simulink model "Drone2_simulink_old"  (R2024b)
settings: Solver=ode1be  StartTime=0.0  StopTime=1200  FixedStep=0.001  MaxStep=0.001  MinStep=0.00095  RelTol=1e-3
undefined symbols (not defined in the file): DiscIntNeverNeededParam, Environment, Newton, Raphson, Sim3dSensor, Vehicle, X, Y, Z
libraries: sm_lib x2953, nesl_utility x76, slpidlib x25, simulink x4, eeGeneralControl x4, matrix_library x3, rllib x2, sim3dlib x2, uavsim3dlib x2, dspstat3 x1, SignalEditorBlockLib x1, sharedutil x1
(part 6 of 21)

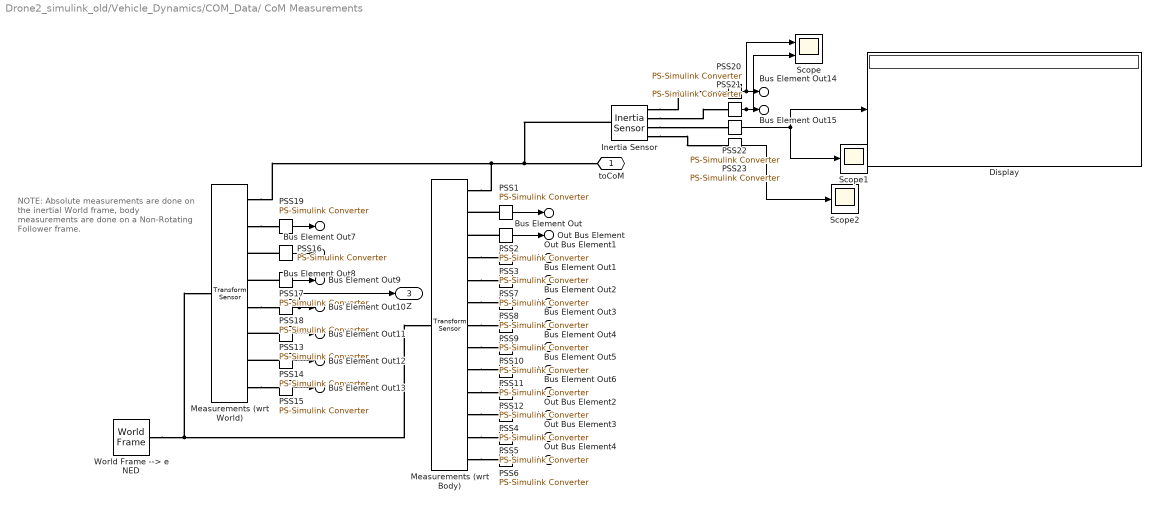
== system Drone2_simulink_old/Vehicle_Dynamics/COM_Data/ CoM Measurements ==
  note: NOTE:
      | Absolute measurements are done on the inertial World frame, body measurements are done on a Non-Rotating Follower frame.
  Display : Display
  Inertia Sensor : sm_lib/Body Elements/Inertia Sensor  SensorExtent=BodyGroup  SpanWeldJoints=off  ExcludeGroundedBodies=off  MeasurementFrame=Attached  SenseMass=on  SenseCenterOfMass=on  SenseInertiaMatrix=on  SenseCenteredInertiaMatrix=off  SensePrincipalInertiaMatrix=on  SenseRotationMatrix=off  GraphicType=PrincipalInertiaFrame  PrincipalInertiaFrameSize=20  GraphicVisPropType=SimpleVisualProperties  GraphicDiffuseColor=[1 0 1]  GraphicOpacity=1  GraphicSpecularColor=[0.5 0.5 0.5 1.0]  GraphicAmbientColor=[0.15 0.15 0.15 1.0]  GraphicEmissiveColor=[0.0 0.0 0.0 1.0]  GraphicShininess=75
  Measurements (wrt Body) : sm_lib/Frames and Transforms/Transform Sensor  MeasurementFrame=NonRotatingFollower  RotationSequence=ZYX  SenseAngle=off  SenseAxis=off  SenseQ=off  SenseR=off  SenseRotationSequence=off  SenseOmegaX=on  SenseOmegaY=on  SenseOmegaZ=on  SenseOmega=off  SenseQDot=off  SenseRDot=off  SenseRotationSequenceDot=off  SenseAlphaX=on  SenseAlphaY=on  SenseAlphaZ=on  SenseAlpha=off  SenseQDDot=off  SenseRDDot=off  SenseX=off  SenseY=off  SenseZ=off  SenseXYZ=off  SenseRad=off  SenseAzim=off  SenseDist=off  SenseInc=off  SenseXDot=on  SenseYDot=on  SenseZDot=on  SenseXYZDot=off  SenseRadDot=off  SenseAzimDot=off  SenseDistDot=off  SenseIncDot=off  SenseXDDot=on  SenseYDDot=on  SenseZDDot=on  SenseXYZDDot=off  SenseRadDDot=off  SenseAzimDDot=off  SenseDistDDot=off  SenseIncDDot=off
  Measurements (wrt World) : sm_lib/Frames and Transforms/Transform Sensor  MeasurementFrame=World  RotationSequence=ZYX  SenseAngle=off  SenseAxis=off  SenseQ=off  SenseR=on  SenseRotationSequence=off  SenseOmegaX=off  SenseOmegaY=off  SenseOmegaZ=off  SenseOmega=off  SenseQDot=off  SenseRDot=off  SenseRotationSequenceDot=off  SenseAlphaX=off  SenseAlphaY=off  SenseAlphaZ=off  SenseAlpha=off  SenseQDDot=off  SenseRDDot=off  SenseX=on  SenseY=on  SenseZ=on  SenseXYZ=off  SenseRad=off  SenseAzim=off  SenseDist=off  SenseInc=off  SenseXDot=on  SenseYDot=on  SenseZDot=on  SenseXYZDot=off  SenseRadDot=off  SenseAzimDot=off  SenseDistDot=off  SenseIncDot=off  SenseXDDot=off  SenseYDDot=off  SenseZDDot=off  SenseXYZDDot=off  SenseRadDDot=off  SenseAzimDDot=off  SenseDistDDot=off  SenseIncDDot=off
  PSS1 : nesl_utility/PS-Simulink Converter  PhysicalDomain=network_engine_domain  SubClassName=ps_output  LeftPortType=input  RightPortType=output  PseudoPeriodic=off  Frequencies=[]  VectorFormat=1-D array  Unit=rad/s  AffineConversion=off
  PSS{10..15} (6 alike) : nesl_utility/PS-Simulink Converter  PhysicalDomain=network_engine_domain  SubClassName=ps_output  LeftPortType=input  RightPortType=output  PseudoPeriodic=off  Frequencies=[]  VectorFormat=1-D array  Unit=m/s  AffineConversion=off
  PSS{16..18,21} (4 alike) : nesl_utility/PS-Simulink Converter  PhysicalDomain=network_engine_domain  SubClassName=ps_output  LeftPortType=input  RightPortType=output  PseudoPeriodic=off  Frequencies=[]  VectorFormat=1-D array  Unit=m  AffineConversion=off
  PSS19 : nesl_utility/PS-Simulink Converter  PhysicalDomain=network_engine_domain  SubClassName=ps_output  LeftPortType=input  RightPortType=output  PseudoPeriodic=off  Frequencies=[]  VectorFormat=1-D array  Unit=1  AffineConversion=off
  PSS2 : nesl_utility/PS-Simulink Converter  PhysicalDomain=network_engine_domain  SubClassName=ps_output  LeftPortType=input  RightPortType=output  PseudoPeriodic=off  Frequencies=[]  VectorFormat=1-D array  Unit=rad/s  AffineConversion=off
  PSS20 : nesl_utility/PS-Simulink Converter  PhysicalDomain=network_engine_domain  SubClassName=ps_output  LeftPortType=input  RightPortType=output  PseudoPeriodic=off  Frequencies=[]  VectorFormat=1-D array  Unit=kg  AffineConversion=off
  PSS22 : nesl_utility/PS-Simulink Converter  PhysicalDomain=network_engine_domain  SubClassName=ps_output  LeftPortType=input  RightPortType=output  PseudoPeriodic=off  Frequencies=[]  VectorFormat=1-D array  Unit=1  AffineConversion=on
  PSS23 : nesl_utility/PS-Simulink Converter  PhysicalDomain=network_engine_domain  SubClassName=ps_output  LeftPortType=input  RightPortType=output  PseudoPeriodic=off  Frequencies=[]  VectorFormat=1-D array  Unit=1  AffineConversion=on
  PSS3 : nesl_utility/PS-Simulink Converter  PhysicalDomain=network_engine_domain  SubClassName=ps_output  LeftPortType=input  RightPortType=output  PseudoPeriodic=off  Frequencies=[]  VectorFormat=1-D array  Unit=rad/s  AffineConversion=off
  PSS4 : nesl_utility/PS-Simulink Converter  PhysicalDomain=network_engine_domain  SubClassName=ps_output  LeftPortType=input  RightPortType=output  PseudoPeriodic=off  Frequencies=[]  VectorFormat=1-D array  Unit=m/s^2  AffineConversion=off
  PSS5 : nesl_utility/PS-Simulink Converter  PhysicalDomain=network_engine_domain  SubClassName=ps_output  LeftPortType=input  RightPortType=output  PseudoPeriodic=off  Frequencies=[]  VectorFormat=1-D array  Unit=m/s^2  AffineConversion=off
  PSS6 : nesl_utility/PS-Simulink Converter  PhysicalDomain=network_engine_domain  SubClassName=ps_output  LeftPortType=input  RightPortType=output  PseudoPeriodic=off  Frequencies=[]  VectorFormat=1-D array  Unit=m/s^2  AffineConversion=off
  PSS7 : nesl_utility/PS-Simulink Converter  PhysicalDomain=network_engine_domain  SubClassName=ps_output  LeftPortType=input  RightPortType=output  PseudoPeriodic=off  Frequencies=[]  VectorFormat=1-D array  Unit=rad/s^2  AffineConversion=off
  PSS8 : nesl_utility/PS-Simulink Converter  PhysicalDomain=network_engine_domain  SubClassName=ps_output  LeftPortType=input  RightPortType=output  PseudoPeriodic=off  Frequencies=[]  VectorFormat=1-D array  Unit=rad/s^2  AffineConversion=off
  PSS9 : nesl_utility/PS-Simulink Converter  PhysicalDomain=network_engine_domain  SubClassName=ps_output  LeftPortType=input  RightPortType=output  PseudoPeriodic=off  Frequencies=[]  VectorFormat=1-D array  Unit=rad/s^2  AffineConversion=off
  Scope : Scope  NumInputPorts=2
  Scope1 : Scope
  Scope2 : Scope
  World Frame --> e NED : sm_lib/Frames and Transforms/World Frame
  toCoM : PMIOPort  Side=Left
  Bus Element Out : Outport  PortName=Body  Element=wb.p
  Out Bus Element : Outport  PortName=Body  Element=wb.q
  Out Bus Element1 : Outport  PortName=Body  Element=wb.r
  Bus Element Out1 : Outport  PortName=Body  Element=dwbdt.pdot
  Bus Element Out2 : Outport  PortName=Body  Element=dwbdt.qdot
  Bus Element Out3 : Outport  PortName=Body  Element=dwbdt.rdot
  Bus Element Out4 : Outport  PortName=Body  Element=Vb.u
  Bus Element Out5 : Outport  PortName=Body  Element=Vb.v
  Bus Element Out6 : Outport  PortName=Body  Element=Vb.w
  Out Bus Element2 : Outport  PortName=Body  Element=Abe.ax
  Out Bus Element3 : Outport  PortName=Body  Element=Abe.ay
  Out Bus Element4 : Outport  PortName=Body  Element=Abe.az
  Bus Element Out14 : Outport  PortName=Body  Element=Mass
  Bus Element Out15 : Outport  PortName=Body  Element=COM
  Bus Element Out7 : Outport  Port=2  PortName=World  Element=R
  Bus Element Out8 : Outport  Port=2  PortName=World  Element=Xe.X
  Bus Element Out9 : Outport  Port=2  PortName=World  Element=Xe.Y
  Bus Element Out10 : Outport  Port=2  PortName=World  Element=Xe.Z
  Bus Element Out11 : Outport  Port=2  PortName=World  Element=Ve.Vx
  Bus Element Out12 : Outport  Port=2  PortName=World  Element=Ve.Vy
  Bus Element Out13 : Outport  Port=2  PortName=World  Element=Ve.Vz
  Z : Outport  Port=3
  wires:
  PSS6/1 -> Out Bus Element4/1
  PSS5/1 -> Out Bus Element3/1
  PSS4/1 -> Out Bus Element2/1
  PSS3/1 -> Out Bus Element1/1
  PSS2/1 -> Out Bus Element/1
  PSS1/1 -> Bus Element Out/1
  PSS8/1 -> Bus Element Out2/1
  PSS9/1 -> Bus Element Out3/1
  PSS10/1 -> Bus Element Out4/1
  PSS11/1 -> Bus Element Out5/1
  PSS12/1 -> Bus Element Out6/1
  PSS13/1 -> Bus Element Out11/1
  PSS14/1 -> Bus Element Out12/1
  PSS15/1 -> Bus Element Out13/1
  PSS16/1 -> Bus Element Out8/1
  PSS18/1 -> Z/1, Bus Element Out10/1
  PSS19/1 -> Bus Element Out7/1
  PSS17/1 -> Bus Element Out9/1
  PSS7/1 -> Bus Element Out1/1
  PSS20/1 -> Scope/1, Bus Element Out14/1
  PSS21/1 -> Scope/2, Bus Element Out15/1
  PSS22/1 -> Scope1/1, Display/1
  PSS23/1 -> Scope2/1
  connections:
  Measurements (wrt Body)/RConn4 -- PSS3/LConn1
  PSS2/LConn1 -- Measurements (wrt Body)/RConn3
  PSS1/LConn1 -- Measurements (wrt Body)/RConn2
  Measurements (wrt Body)/RConn1 -- Measurements (wrt World)/RConn1 -- Inertia Sensor/LConn1 -- toCoM/RConn1
  World Frame --> e NED/RConn1 -- Measurements (wrt World)/LConn1 -- Measurements (wrt Body)/LConn1
  Measurements (wrt Body)/RConn11 -- PSS4/LConn1
  Measurements (wrt Body)/RConn12 -- PSS5/LConn1
  Measurements (wrt Body)/RConn13 -- PSS6/LConn1
  Measurements (wrt Body)/RConn5 -- PSS7/LConn1
  Measurements (wrt Body)/RConn6 -- PSS8/LConn1
  Measurements (wrt Body)/RConn7 -- PSS9/LConn1
  Measurements (wrt Body)/RConn8 -- PSS10/LConn1
  Measurements (wrt Body)/RConn9 -- PSS11/LConn1
  Measurements (wrt Body)/RConn10 -- PSS12/LConn1
  PSS13/LConn1 -- Measurements (wrt World)/RConn6
  PSS14/LConn1 -- Measurements (wrt World)/RConn7
  Measurements (wrt World)/RConn8 -- PSS15/LConn1
  PSS16/LConn1 -- Measurements (wrt World)/RConn3
  PSS17/LConn1 -- Measurements (wrt World)/RConn4
  Measurements (wrt World)/RConn5 -- PSS18/LConn1
  Measurements (wrt World)/RConn2 -- PSS19/LConn1
  Inertia Sensor/RConn1 -- PSS20/LConn1
  Inertia Sensor/RConn2 -- PSS21/LConn1
  Inertia Sensor/RConn3 -- PSS22/LConn1
  Inertia Sensor/RConn4 -- PSS23/LConn1

== system Drone2_simulink_old/Vehicle_Dynamics/COM_Data/Derived Measurements ==
  Bus Element In1 : Inport  PortName=Body  Element=wb
  Bus Element In2 : Inport  PortName=Body  Element=Vb
  Bus Element In3 : Inport  PortName=Body  Element=Abe
  Bus Element In : Inport  Port=2  PortName=World  Element=R
  Body Acceleration : Subsystem
  Calculate DCM : Subsystem
  Euler Angles : Subsystem
  Incidence Angles : Subsystem
  Bus Element Out1 : Outport  PortName=Derived  Element=Euler.phi
  Bus Element Out2 : Outport  PortName=Derived  Element=Euler.theta
  Bus Element Out3 : Outport  PortName=Derived  Element=Euler.psi
  Bus Element Out4 : Outport  PortName=Derived  Element=Body.Abb
  Bus Element Out7 : Outport  PortName=Derived  Element=Body.V
  Bus Element Out5 : Outport  PortName=Derived  Element=Body.Incidences.alpha
  Bus Element Out6 : Outport  PortName=Derived  Element=Body.Incidences.beta
  Bus Element Out : Outport  PortName=Derived  Element=World.DCMbe
  wires:
  Bus Element In1/1 -> Euler Angles/1(pqr), Body Acceleration/1(wb)
  Euler Angles/1(phi) -> Bus Element Out1/1
  Euler Angles/2(theta) -> Bus Element Out2/1
  Euler Angles/3(psi) -> Bus Element Out3/1
  Bus Element In/1 -> Calculate DCM/1(R)
  Calculate DCM/1(DCMbe) -> Bus Element Out/1
  Bus Element In2/1 -> Incidence Angles/1(Vb), Body Acceleration/2(Vb)
  Bus Element In3/1 -> Body Acceleration/3(Abe)
  Incidence Angles/1(alpha) -> Bus Element Out5/1
  Incidence Angles/2(beta) -> Bus Element Out6/1
  Incidence Angles/3(V) -> Bus Element Out7/1
  Body Acceleration/1(Abb) -> Bus Element Out4/1

== system Drone2_simulink_old/Vehicle_Dynamics/Drone_Assembly/Arm Assembly ==
  Bus Element In : Inport  PortName=Aerial  Element=MotorRB
  Bus Element In1 : Inport  PortName=Aerial  Element=MotorRF
  Bus Element In2 : Inport  PortName=Aerial  Element=MotorLB
  Bus Element In3 : Inport  PortName=Aerial  Element=MotorLF
  ArmMotor : Subsystem
      settings: PortSchema="{\"entries\":[{\"content\":{\"sides\":[{\"content\":{\"connectorIds\":[\"LConn1\",\"LConn2\"]},\"type\":\"ConnectorPlacement.EquallySpacedRectSide\",\"uuid\":\"18c07681-30da-4c28-9f47-7bd1e0aa44ed\"},{\"content\":{\"connectorIds\":[\"RConn1\",\"RConn2\"],\"side\":\"RIGHT\"},\"type\":\"ConnectorPlacement.EquallySpacedRectSide\",\"uuid\":\"06a64526-1d01-4100-b1c2-518ccd3ce88b\"},{\"content\":{\"side\":\"TOP\"},\"type\":\"ConnectorPlacement.EquallySpacedRectSide\",\"uuid\":\"c35bb6b8-7cf8-44c8-8640-006f8f005921\"},{\"content\":{\"connectorIds\":[\"RConn3\"],\"side\":\"BOTTOM\"},\"type\":\"ConnectorPlacement.EquallySpacedRectSide\",\"uuid\":\"7c66519b-fd2c-4113-b0b7-4af298a3d539\"}]},\"type\":\"ConnectorPlacement.EquallySpacedConnector\",\"uuid\":\"9b76760e-a410-492a-8101-e92960cefc09\"}],\"packageUris\":[\"http://schema.mathworks.com/mf0/Connector/R2020b\"],\"version\":\"1.0\"}"
  Bottomplate : sm_lib/Body Elements/File Solid  ExtGeomFileName=outersupportPlate.STL  UnitType=Custom  ExtGeomFileUnits=mm  StepReaderType=HEX  ExportConvexHullGeometry=off  InertiaType=CalculateFromGeometry  BasedOnType=Density  Density=1000  DensityUnits=kg/m^3  Mass=1  MassUnits=kg  CenterOfMass=[0 0 0]  CenterOfMassUnits=m  MomentsOfInertia=[1 1 1]  MomentsOfInertiaUnits=kg*m^2  ProductsOfInertia=[0 0 0]  ProductsOfInertiaUnits=kg*m^2  GraphicType=None  MarkerShape=Sphere  MarkerSize=10  GraphicVisPropType=SimpleVisualProperties  GraphicDiffuseColor=[0.5 0.5 0.5]  GraphicOpacity=1  GraphicSpecularColor=[0.5 0.5 0.5 1.0]  GraphicAmbientColor=[0.15 0.15 0.15 1.0]  GraphicEmissiveColor=[0.0 0.0 0.0 1.0]  GraphicShininess=75  DoExposeReferenceFrame=on  SerializedFrames=<Frames/>
  ForceTorqueP1 : Subsystem  mask{Min_Thrust=0, Max_Thrust=Vehicle.Motor.MaxThrust, Min_torque=0, Max_torque=Vehicle.Motor.Maxtorque, Gain=CCW}
      mask prompts: Min_Thrust "Min Force"; Max_Thrust "Max Force"; Min_torque "Min Torque"; Max_torque "Max Torque"; Gain "Rotatiopn"
      settings: PortSchema="{\"entries\":[{\"content\":{\"sides\":[{\"content\":{\"connectorIds\":[\"LConn1\",\"In1\"]},\"type\":\"ConnectorPlacement.EquallySpacedRectSide\",\"uuid\":\"ffafe241-07d7-43e0-ae4d-643c4a08182f\"},{\"content\":{\"connectorIds\":[\"RConn1\"],\"side\":\"RIGHT\"},\"type\":\"ConnectorPlacement.EquallySpacedRectSide\",\"uuid\":\"ab03b775-9680-440b-91a4-d2ad69d05908\"},{\"content\":{\"side\":\"TOP\"},\"type\":\"ConnectorPlacement.EquallySpacedRectSide\",\"uuid\":\"9b5f7a56-64a3-4e6c-951e-4d16d9e86562\"}]},\"type\":\"ConnectorPlacement.EquallySpacedConnector\",\"uuid\":\"60e02493-35c3-4a07-9d64-09ca7aed531f\"}],\"packageUris\":[\"http://schema.mathworks.com/mf0/Connector/R2020b\"],\"version\":\"1.0\"}"
      mask DialogControl Container4 Prompt: Force
      mask DialogControl Container5 Prompt: Torque
  ForceTorqueP2 : Subsystem  mask{Min_Thrust=0, Max_Thrust=Vehicle.Motor.MaxThrust, Min_torque=0, Max_torque=Vehicle.Motor.Maxtorque, Gain=CW}
      mask prompts: Min_Thrust "Min Force"; Max_Thrust "Max Force"; Min_torque "Min Torque"; Max_torque "Max Torque"; Gain "Rotatiopn"
      settings: PortSchema="{\"entries\":[{\"content\":{\"sides\":[{\"content\":{\"connectorIds\":[\"LConn1\",\"In1\"]},\"type\":\"ConnectorPlacement.EquallySpacedRectSide\",\"uuid\":\"ffafe241-07d7-43e0-ae4d-643c4a08182f\"},{\"content\":{\"connectorIds\":[\"RConn1\"],\"side\":\"RIGHT\"},\"type\":\"ConnectorPlacement.EquallySpacedRectSide\",\"uuid\":\"ab03b775-9680-440b-91a4-d2ad69d05908\"},{\"content\":{\"side\":\"TOP\"},\"type\":\"ConnectorPlacement.EquallySpacedRectSide\",\"uuid\":\"9b5f7a56-64a3-4e6c-951e-4d16d9e86562\"}]},\"type\":\"ConnectorPlacement.EquallySpacedConnector\",\"uuid\":\"60e02493-35c3-4a07-9d64-09ca7aed531f\"}],\"packageUris\":[\"http://schema.mathworks.com/mf0/Connector/R2020b\"],\"version\":\"1.0\"}"
      mask DialogControl Container4 Prompt: Force
      mask DialogControl Container5 Prompt: Torque
  ForceTorqueP3 : Subsystem  mask{Min_Thrust=0, Max_Thrust=Vehicle.Motor.MaxThrust, Min_torque=0, Max_torque=Vehicle.Motor.Maxtorque, Gain=CCW}
      mask prompts: Min_Thrust "Min Force"; Max_Thrust "Max Force"; Min_torque "Min Torque"; Max_torque "Max Torque"; Gain "Rotatiopn"
      settings: PortSchema="{\"entries\":[{\"content\":{\"sides\":[{\"content\":{\"connectorIds\":[\"LConn1\",\"In1\"]},\"type\":\"ConnectorPlacement.EquallySpacedRectSide\",\"uuid\":\"ffafe241-07d7-43e0-ae4d-643c4a08182f\"},{\"content\":{\"connectorIds\":[\"RConn1\"],\"side\":\"RIGHT\"},\"type\":\"ConnectorPlacement.EquallySpacedRectSide\",\"uuid\":\"ab03b775-9680-440b-91a4-d2ad69d05908\"},{\"content\":{\"side\":\"TOP\"},\"type\":\"ConnectorPlacement.EquallySpacedRectSide\",\"uuid\":\"9b5f7a56-64a3-4e6c-951e-4d16d9e86562\"}]},\"type\":\"ConnectorPlacement.EquallySpacedConnector\",\"uuid\":\"60e02493-35c3-4a07-9d64-09ca7aed531f\"}],\"packageUris\":[\"http://schema.mathworks.com/mf0/Connector/R2020b\"],\"version\":\"1.0\"}"
      mask DialogControl Container4 Prompt: Force
      mask DialogControl Container5 Prompt: Torque
  ForceTorqueP4 : Subsystem  mask{Min_Thrust=0, Max_Thrust=Vehicle.Motor.MaxThrust, Min_torque=0, Max_torque=Vehicle.Motor.Maxtorque, Gain=CW}
      mask prompts: Min_Thrust "Min Force"; Max_Thrust "Max Force"; Min_torque "Min Torque"; Max_torque "Max Torque"; Gain "Rotatiopn"
      settings: PortSchema="{\"entries\":[{\"content\":{\"sides\":[{\"content\":{\"connectorIds\":[\"LConn1\",\"In1\"]},\"type\":\"ConnectorPlacement.EquallySpacedRectSide\",\"uuid\":\"ffafe241-07d7-43e0-ae4d-643c4a08182f\"},{\"content\":{\"connectorIds\":[\"RConn1\"],\"side\":\"RIGHT\"},\"type\":\"ConnectorPlacement.EquallySpacedRectSide\",\"uuid\":\"ab03b775-9680-440b-91a4-d2ad69d05908\"},{\"content\":{\"side\":\"TOP\"},\"type\":\"ConnectorPlacement.EquallySpacedRectSide\",\"uuid\":\"9b5f7a56-64a3-4e6c-951e-4d16d9e86562\"}]},\"type\":\"ConnectorPlacement.EquallySpacedConnector\",\"uuid\":\"60e02493-35c3-4a07-9d64-09ca7aed531f\"}],\"packageUris\":[\"http://schema.mathworks.com/mf0/Connector/R2020b\"],\"version\":\"1.0\"}"
      mask DialogControl Container4 Prompt: Force
      mask DialogControl Container5 Prompt: Torque
  Landing gear : Subsystem
  M8Nutbolat on plates : Subsystem
  Prop{1..4} (4 alike) : sm_lib/Body Elements/File Solid  ExtGeomFileName=10x4.5L.STL  UnitType=Custom  ExtGeomFileUnits=mm  StepReaderType=HEX  ExportConvexHullGeometry=off  InertiaType=CalculateFromGeometry  BasedOnType=Density  Density=940  DensityUnits=kg/m^3  Mass=1  MassUnits=kg  CenterOfMass=[0 0 0]  CenterOfMassUnits=m  MomentsOfInertia=[1 1 1]  MomentsOfInertiaUnits=kg*m^2  ProductsOfInertia=[0 0 0]  ProductsOfInertiaUnits=kg*m^2  GraphicType=None  MarkerShape=Sphere  MarkerSize=10  GraphicVisPropType=SimpleVisualProperties  GraphicDiffuseColor=[0.2 0.2 1.0]  GraphicOpacity=1  GraphicSpecularColor=[0.5 0.5 0.5 1.0]  GraphicAmbientColor=[0.15 0.15 0.15 1.0]  GraphicEmissiveColor=[0.0 0.0 0.0 1.0]  GraphicShininess=75  DoExposeReferenceFrame=off  SerializedFrames=<Frames><Frame><Id>Frame1</Id><Value><Name>R</Name><Origin><Source>CenterOfMassFrame</Source><FeatureName></FeatureName></Origin><PrimaryAxis><DefinedDirection>+Z</DefinedDirection><Source>ReferenceFrame</Source><SourceDirection>+Y</SourceDirection><FeatureName></FeatureName></PrimaryAxis><SecondaryAxis><DefinedDirection>+X</DefinedDirection><Source>ReferenceFrame</Source><SourceDirection>+X</SourceDirection><FeatureName></FeatureName></SecondaryAxis></Value></Frame></Frames>
  TopPlatetoFirstHole : sm_lib/Frames and Transforms/Rigid Transform  RotationMethod=None  FollAlignAxisA=+X  BaseAlignAxisA=+Y  FollAlignAxisB=+Y  BaseAlignAxisB=+Z  RotationStandardAxis=+Z  RotationAngle=0  RotationAngleUnits=deg  RotationArbitraryAxis=[0 0 1]  RotationSequenceAxes=FollowerAxes  RotationSequence=XYX  RotationSequenceAngles=[0 0 0]  RotationSequenceAnglesUnits=deg  RotationMatrix=[1 0 0;0 1 0;0 0 1]  Quaternion=[1 0 0 0]  TranslationMethod=Cartesian  TranslationCartesianOffset=[0.015 0.012 0.06125]  TranslationCartesianOffsetUnits=m  TranslationStandardAxis=+Z  TranslationStandardOffset=0  TranslationStandardOffsetUnits=m  TranslationROffset=0  TranslationROffsetUnits=m  TranslationThetaOffset=0  TranslationThetaOffsetUnits=deg  TranslationZOffset=0  TranslationZOffsetUnits=m
  Topplate : sm_lib/Body Elements/File Solid  ExtGeomFileName=outersupportPlate.STL  UnitType=Custom  ExtGeomFileUnits=mm  StepReaderType=HEX  ExportConvexHullGeometry=off  InertiaType=CalculateFromGeometry  BasedOnType=Density  Density=1000  DensityUnits=kg/m^3  Mass=1  MassUnits=kg  CenterOfMass=[0 0 0]  CenterOfMassUnits=m  MomentsOfInertia=[1 1 1]  MomentsOfInertiaUnits=kg*m^2  ProductsOfInertia=[0 0 0]  ProductsOfInertiaUnits=kg*m^2  GraphicType=FromGeometry  MarkerShape=Sphere  MarkerSize=10  GraphicVisPropType=SimpleVisualProperties  GraphicDiffuseColor=[0.5 0.5 0.5]  GraphicOpacity=1  GraphicSpecularColor=[0.5 0.5 0.5 1.0]  GraphicAmbientColor=[0.15 0.15 0.15 1.0]  GraphicEmissiveColor=[0.0 0.0 0.0 1.0]  GraphicShininess=75  DoExposeReferenceFrame=on  SerializedFrames=<Frames/>
  centertoBottomplate1 : sm_lib/Frames and Transforms/Rigid Transform  RotationMethod=AlignedAxes  FollAlignAxisA=+X  BaseAlignAxisA=+X  FollAlignAxisB=-Z  BaseAlignAxisB=+Z  RotationStandardAxis=+Z  RotationAngle=0  RotationAngleUnits=deg  RotationArbitraryAxis=[0 0 1]  RotationSequenceAxes=FollowerAxes  RotationSequence=XYX  RotationSequenceAngles=[0 0 0]  RotationSequenceAnglesUnits=deg  RotationMatrix=[1 0 0;0 1 0;0 0 1]  Quaternion=[1 0 0 0]  TranslationMethod=Cartesian  TranslationCartesianOffset=[-0.2425 0.100 0]  TranslationCartesianOffsetUnits=m  TranslationStandardAxis=+Z  TranslationStandardOffset=0  TranslationStandardOffsetUnits=m  TranslationROffset=0  TranslationROffsetUnits=m  TranslationThetaOffset=0  TranslationThetaOffsetUnits=deg  TranslationZOffset=0  TranslationZOffsetUnits=m
  centertoTopplate : sm_lib/Frames and Transforms/Rigid Transform  RotationMethod=None  FollAlignAxisA=+X  BaseAlignAxisA=+Y  FollAlignAxisB=+Y  BaseAlignAxisB=+Z  RotationStandardAxis=+Z  RotationAngle=0  RotationAngleUnits=deg  RotationArbitraryAxis=[0 0 1]  RotationSequenceAxes=FollowerAxes  RotationSequence=XYX  RotationSequenceAngles=[0 0 0]  RotationSequenceAnglesUnits=deg  RotationMatrix=[1 0 0;0 1 0;0 0 1]  Quaternion=[1 0 0 0]  TranslationMethod=Cartesian  TranslationCartesianOffset=[-0.2425 -0.100 0]  TranslationCartesianOffsetUnits=m  TranslationStandardAxis=+Z  TranslationStandardOffset=0  TranslationStandardOffsetUnits=m  TranslationROffset=0  TranslationROffsetUnits=m  TranslationThetaOffset=0  TranslationThetaOffsetUnits=deg  TranslationZOffset=0  TranslationZOffsetUnits=m
  From CO : PMIOPort  Side=Right
  wires:
  Bus Element In/1 -> ForceTorqueP1/1(MotorRB)
  Bus Element In1/1 -> ForceTorqueP2/1(MotorRF)
  Bus Element In2/1 -> ForceTorqueP4/1(MotorLB)
  Bus Element In3/1 -> ForceTorqueP3/1(MotorLF)
  connections:
  From CO/RConn1 -- centertoTopplate/LConn1 -- centertoBottomplate1/LConn1
  centertoBottomplate1/RConn1 -- Bottomplate/RConn1
  TopPlatetoFirstHole/RConn1 -- M8Nutbolat on plates/LConn1
  ForceTorqueP1/RConn1 -- ArmMotor/LConn1
  Prop1/LConn1 -- ForceTorqueP1/LConn1
  ForceTorqueP2/RConn1 -- ArmMotor/LConn2
  ForceTorqueP2/LConn1 -- Prop2/LConn1
  ForceTorqueP3/LConn1 -- Prop3/LConn1
  ForceTorqueP3/RConn1 -- ArmMotor/RConn2
  ForceTorqueP4/RConn1 -- ArmMotor/RConn1
  Prop4/LConn1 -- ForceTorqueP4/LConn1
  TopPlatetoFirstHole/LConn1 -- Landing gear/RConn1 -- ArmMotor/RConn3 -- Topplate/RConn1 -- centertoTopplate/RConn1

== system Drone2_simulink_old/Vehicle_Dynamics/Drone_Assembly/Cylinder_Assembly ==
  Force : Inport
  AcrPlate : sm_lib/Body Elements/File Solid  ExtGeomFileName=Plate.STL  UnitType=Custom  ExtGeomFileUnits=mm  StepReaderType=HEX  ExportConvexHullGeometry=off  InertiaType=CalculateFromGeometry  BasedOnType=Density  Density=1200  DensityUnits=kg/m^3  Mass=1  MassUnits=kg  CenterOfMass=[0 0 0]  CenterOfMassUnits=m  MomentsOfInertia=[1 1 1]  MomentsOfInertiaUnits=kg*m^2  ProductsOfInertia=[0 0 0]  ProductsOfInertiaUnits=kg*m^2  GraphicType=FromGeometry  MarkerShape=Sphere  MarkerSize=10  GraphicVisPropType=SimpleVisualProperties  GraphicDiffuseColor=[0.5 0.5 0.5]  GraphicOpacity=1  GraphicSpecularColor=[0.5 0.5 0.5 1.0]  GraphicAmbientColor=[0.15 0.15 0.15 1.0]  GraphicEmissiveColor=[0.0 0.0 0.0 1.0]  GraphicShininess=75  DoExposeReferenceFrame=on  SerializedFrames=<Frames/>
  BackCap : Subsystem
      settings: PortSchema="{\"entries\":[{\"content\":{\"sides\":[{\"content\":{},\"type\":\"ConnectorPlacement.EquallySpacedRectSide\",\"uuid\":\"6d84b478-2856-425e-8b15-5b8c768f2c45\"},{\"content\":{\"side\":\"RIGHT\"},\"type\":\"ConnectorPlacement.EquallySpacedRectSide\",\"uuid\":\"90d7fc9f-942c-41ea-87e8-f98ad4c8ee77\"},{\"content\":{\"connectorIds\":[\"LConn1\"],\"side\":\"TOP\"},\"type\":\"ConnectorPlacement.EquallySpacedRectSide\",\"uuid\":\"597fe308-f5c8-431e-a4a8-973ffab3114b\"}]},\"type\":\"ConnectorPlacement.EquallySpacedConnector\",\"uuid\":\"7d64c5eb-ad59-4e7e-9aa7-9e749246dabe\"}],\"packageUris\":[\"http://schema.mathworks.com/mf0/Connector/R2020b\"],\"version\":\"1.0\"}"
      mask Display: image('Cap_Subsystem.PNG');
  Below_Plate_batery and sensors : Subsystem
      settings: PortSchema="{\"entries\":[{\"content\":{\"sides\":[{\"content\":{},\"type\":\"ConnectorPlacement.EquallySpacedRectSide\",\"uuid\":\"6d84b478-2856-425e-8b15-5b8c768f2c45\"},{\"content\":{\"side\":\"RIGHT\"},\"type\":\"ConnectorPlacement.EquallySpacedRectSide\",\"uuid\":\"90d7fc9f-942c-41ea-87e8-f98ad4c8ee77\"},{\"content\":{\"connectorIds\":[\"LConn1\"],\"side\":\"TOP\"},\"type\":\"ConnectorPlacement.EquallySpacedRectSide\",\"uuid\":\"597fe308-f5c8-431e-a4a8-973ffab3114b\"}]},\"type\":\"ConnectorPlacement.EquallySpacedConnector\",\"uuid\":\"7d64c5eb-ad59-4e7e-9aa7-9e749246dabe\"}],\"packageUris\":[\"http://schema.mathworks.com/mf0/Connector/R2020b\"],\"version\":\"1.0\"}"
  BuoyancySystem : Subsystem
      settings: PortSchema="{\"entries\":[{\"content\":{\"sides\":[{\"content\":{\"connectorIds\":[\"In1\"]},\"type\":\"ConnectorPlacement.EquallySpacedRectSide\",\"uuid\":\"da56b2fd-2863-460f-b4f6-53390ff3aaae\"},{\"content\":{\"connectorIds\":[\"Out1\"],\"side\":\"RIGHT\"},\"type\":\"ConnectorPlacement.EquallySpacedRectSide\",\"uuid\":\"028912b2-1aa2-4953-8029-051f1e961216\"},{\"content\":{\"connectorIds\":[\"LConn1\",\"LConn2\",\"LConn3\",\"LConn4\"],\"side\":\"TOP\"},\"type\":\"ConnectorPlacement.EquallySpacedRectSide\",\"uuid\":\"9f3556d9-d00a-4abf-97e1-d4fc3f654490\"}]},\"type\":\"ConnectorPlacement.EquallySpacedConnector\",\"uuid\":\"3db711f2-b116-4a03-bbed-aba615cd386f\"}],\"packageUris\":[\"http://schema.mathworks.com/mf0/Connector/R2020b\"],\"version\":\"1.0\"}"
      mask Display: image('buoyancysystem.PNG');
  CentretoPlate : sm_lib/Frames and Transforms/Rigid Transform  RotationMethod=StandardAxis  FollAlignAxisA=+X  BaseAlignAxisA=+X  FollAlignAxisB=+Y  BaseAlignAxisB=-Y  RotationStandardAxis=+X  RotationAngle=-90  RotationAngleUnits=deg  RotationArbitraryAxis=[0 0 1]  RotationSequenceAxes=FollowerAxes  RotationSequence=XYX  RotationSequenceAngles=[0 0 0]  RotationSequenceAnglesUnits=deg  RotationMatrix=[1 0 0;0 1 0;0 0 1]  Quaternion=[1 0 0 0]  TranslationMethod=Cartesian  TranslationCartesianOffset=[-0.213 -0.07445 0.007]  TranslationCartesianOffsetUnits=m  TranslationStandardAxis=+Z  TranslationStandardOffset=0  TranslationStandardOffsetUnits=m  TranslationROffset=0  TranslationROffsetUnits=m  TranslationThetaOffset=0  TranslationThetaOffsetUnits=deg  TranslationZOffset=0  TranslationZOffsetUnits=m
  Cylinder : sm_lib/Body Elements/File Solid  ExtGeomFileName=cylinderical_body.stl  UnitType=Custom  ExtGeomFileUnits=mm  StepReaderType=HEX  ExportConvexHullGeometry=on  InertiaType=CalculateFromGeometry  BasedOnType=Density  Density=1200  DensityUnits=kg/m^3  Mass=1.3418  MassUnits=kg  CenterOfMass=[0.225 0.08 0.08]  CenterOfMassUnits=m  MomentsOfInertia=[0.0079 0.0261 0.0261]  MomentsOfInertiaUnits=kg*m^2  ProductsOfInertia=[0 0 0]  ProductsOfInertiaUnits=kg*m^2  GraphicType=None  MarkerShape=Sphere  MarkerSize=10  GraphicVisPropType=SimpleVisualProperties  GraphicDiffuseColor=[1.0 0.0 0.8]  GraphicOpacity=0.1  GraphicSpecularColor=[0.5 0.5 0.5 1.0]  GraphicAmbientColor=[0.15 0.15 0.15 1.0]  GraphicEmissiveColor=[0.0 0.0 0.0 1.0]  GraphicShininess=75  DoExposeReferenceFrame=on  SerializedFrames=<Frames/>
  CylindertoCentre : sm_lib/Frames and Transforms/Rigid Transform  RotationMethod=None  FollAlignAxisA=+X  BaseAlignAxisA=+Y  FollAlignAxisB=+Y  BaseAlignAxisB=+Z  RotationStandardAxis=+Z  RotationAngle=0  RotationAngleUnits=deg  RotationArbitraryAxis=[0 0 1]  RotationSequenceAxes=FollowerAxes  RotationSequence=XYX  RotationSequenceAngles=[0 0 0]  RotationSequenceAnglesUnits=deg  RotationMatrix=[1 0 0;0 1 0;0 0 1]  Quaternion=[1 0 0 0]  TranslationMethod=Cartesian  TranslationCartesianOffset=[0.225 0.0808 0.080839]  TranslationCartesianOffsetUnits=m  TranslationStandardAxis=+Z  TranslationStandardOffset=0  TranslationStandardOffsetUnits=m  TranslationROffset=0  TranslationROffsetUnits=m  TranslationThetaOffset=0  TranslationThetaOffsetUnits=deg  TranslationZOffset=0  TranslationZOffsetUnits=m
  Frontcap : Subsystem
      settings: PortSchema="{\"entries\":[{\"content\":{\"sides\":[{\"content\":{},\"type\":\"ConnectorPlacement.EquallySpacedRectSide\",\"uuid\":\"6d84b478-2856-425e-8b15-5b8c768f2c45\"},{\"content\":{\"side\":\"RIGHT\"},\"type\":\"ConnectorPlacement.EquallySpacedRectSide\",\"uuid\":\"90d7fc9f-942c-41ea-87e8-f98ad4c8ee77\"},{\"content\":{\"connectorIds\":[\"LConn1\"],\"side\":\"TOP\"},\"type\":\"ConnectorPlacement.EquallySpacedRectSide\",\"uuid\":\"597fe308-f5c8-431e-a4a8-973ffab3114b\"}]},\"type\":\"ConnectorPlacement.EquallySpacedConnector\",\"uuid\":\"7d64c5eb-ad59-4e7e-9aa7-9e749246dabe\"}],\"packageUris\":[\"http://schema.mathworks.com/mf0/Connector/R2020b\"],\"version\":\"1.0\"}"
      mask Display: image('Cap_Subsystem.PNG');
  origin to cylinderLLC : sm_lib/Frames and Transforms/Rigid Transform  RotationMethod=None  FollAlignAxisA=+X  BaseAlignAxisA=+Y  FollAlignAxisB=+Y  BaseAlignAxisB=+Z  RotationStandardAxis=+Z  RotationAngle=0  RotationAngleUnits=deg  RotationArbitraryAxis=[0 0 1]  RotationSequenceAxes=FollowerAxes  RotationSequence=XYX  RotationSequenceAngles=[0 0 0]  RotationSequenceAnglesUnits=deg  RotationMatrix=[1 0 0;0 1 0;0 0 1]  Quaternion=[1 0 0 0]  TranslationMethod=Cartesian  TranslationCartesianOffset=[-0.225 -0.080 -0.080]  TranslationCartesianOffsetUnits=m  TranslationStandardAxis=+Z  TranslationStandardOffset=0  TranslationStandardOffsetUnits=m  TranslationROffset=0  TranslationROffsetUnits=m  TranslationThetaOffset=0  TranslationThetaOffsetUnits=deg  TranslationZOffset=0  TranslationZOffsetUnits=m
  FromCO : PMIOPort  Side=Left
  Cylinderhull : PMIOPort  Port=2  Side=Left
  FL : PMIOPort  Port=3  Side=Left
  FR : PMIOPort  Port=4  Side=Left
  R : PMIOPort  Port=5  Side=Left
  Out Bus Element : Outport  PortName=Buoyancy  Element=Syringe
  wires:
  BuoyancySystem/1(Syringe) -> Out Bus Element/1
  Force/1 -> BuoyancySystem/1(Force)
  connections:
  Cylinder/RConn1 -- origin to cylinderLLC/RConn1 -- CylindertoCentre/LConn1
  CylindertoCentre/RConn1 -- CentretoPlate/LConn1 -- Frontcap/LConn1 -- BackCap/LConn1 -- Below_Plate_batery and sensors/LConn1 -- BuoyancySystem/LConn1
  origin to cylinderLLC/LConn1 -- FromCO/RConn1
  AcrPlate/RConn1 -- CentretoPlate/RConn1
  Cylinderhull/RConn1 -- Cylinder/LConn1
  FR/RConn1 -- BuoyancySystem/LConn2
  FL/RConn1 -- BuoyancySystem/LConn3
  R/RConn1 -- BuoyancySystem/LConn4
